simulink subsystem "EngineBasic_refsub"  (R2022a)
settings: Solver=VariableStepAuto  StartTime=0.0  StopTime=10.0  RelTol=1e-3
undefined symbols (not defined in the file): engine
libraries: fl_lib x11, nesl_utility x2, sdl_lib x1
settings Model: Creator=isaacito  LastModifiedBy=isaacito
settings SolverCC: AlgebraicLoopSolver=TrustRegion
settings DebuggingCC: UnconnectedInputMsg=warning  UnconnectedOutputMsg=warning  UnconnectedLineMsg=warning  SFMachineParentedDataDiag=warning
settings RTWCC: DLArmComputeVersion=19.05

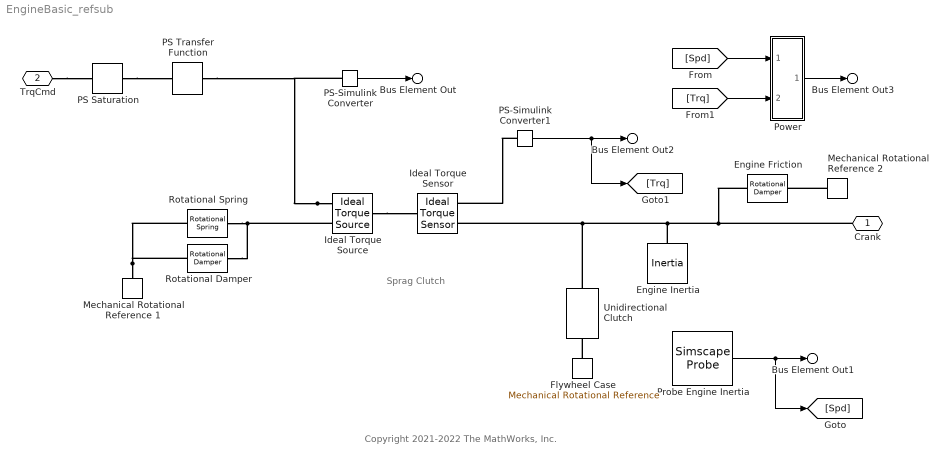
== system EngineBasic_refsub ==
  note: Copyright 2021-2022 The MathWorks, Inc.
  note: Sprag Clutch
  Engine Friction : fl_lib/Mechanical/Rotational Elements/Rotational Damper  D=engine.damping_Nm_per_rpm m*N/rpm  w_specify=off  w_priority=None  w=0 rad/s  w_nominal_specify=off  w_nominal_unit=rad/s  w_nominal_value=1  t_specify=off  t_priority=None  t=0 N*m  t_nominal_specify=off  t_nominal_unit=N*m  t_nominal_value=1
      settings: SourceProductBaseCode=PW,SS,VE
  Engine Inertia : fl_lib/Mechanical/Rotational Elements/Inertia  inertia=engine.inertia_kg_m2 kg*m^2  num_ports=foundation.enum.numPorts2.one  w_specify=on  w_priority=None  w=initial.engine_speed_rpm rpm  w_nominal_specify=off  w_nominal_unit=rad/s  w_nominal_value=1  t_specify=off  t_priority=None  t=0 N*m  t_nominal_specify=off  t_nominal_unit=N*m  t_nominal_value=1
      settings: SourceProductBaseCode=PW,SS,VE
      settings: AttributesFormatString=|
      | %<inertia> (%<inertia_unit>)
      | %<w> (%<w_unit>)
      | Priority: %<w_priority>
  Flywheel Case : fl_lib/Mechanical/Rotational Elements/Mechanical Rotational Reference
      settings: SourceProductBaseCode=PW,SS,VE
  Ideal Torque Sensor : fl_lib/Mechanical/Mechanical Sensors/Ideal Torque Sensor
      settings: SourceProductBaseCode=PW,SS,VE
  Ideal Torque Source : fl_lib/Mechanical/Mechanical Sources/Ideal Torque Source
      settings: SourceProductBaseCode=PW,SS,VE
  Mechanical Rotational Reference 1 : fl_lib/Mechanical/Rotational Elements/Mechanical Rotational Reference
      settings: SourceProductBaseCode=PW,SS,VE
  Mechanical Rotational Reference 2 : fl_lib/Mechanical/Rotational Elements/Mechanical Rotational Reference
      settings: SourceProductBaseCode=PW,SS,VE
  PS Saturation : fl_lib/Physical Signals/Nonlinear Operators/PS Saturation  upper_limit=engine.trqMax_Nm N*m  lower_limit=0 N*m
      settings: AttributesFormatString=%<upper_limit> (%<upper_limit_unit>)  SourceProductBaseCode=PW,SS,VE
  PS Transfer Function : fl_lib/Physical Signals/Linear Operators/PS Transfer Function  transfer_function_type=foundation.enum.transfer_function_type.lag  T=engine.lag_s s  T1=2 s  T2=1 s  y0=initial.engine_torque_Nm N*m
      settings: SourceProductBaseCode=PW,SS,VE  InternalSimscapePortConfiguration="{\"Bottom\":[],\"Left\":[{\"id\":\"U\",\"label\":\"\",\"type\":\"input\"}],\"Right\":[{\"id\":\"Y\",\"label\":\"\",\"type\":\"output\"}],\"Top\":[]}"
      settings: AttributesFormatString=|
      | %<T> [%<T_unit>]
      | Initial: %<y0> [%<y0_unit>]
  PS-Simulink Converter : nesl_utility/PS-Simulink Converter  PhysicalDomain=network_engine_domain  SubClassName=ps_output  LeftPortType=input  RightPortType=output  PseudoPeriodic=off  Frequencies=[]  VectorFormat=1-D array  Unit=N*m  AffineConversion=off
      settings: SourceProductBaseCode=SS,PW,VE
  PS-Simulink Converter1 : nesl_utility/PS-Simulink Converter  PhysicalDomain=network_engine_domain  SubClassName=ps_output  LeftPortType=input  RightPortType=output  PseudoPeriodic=off  Frequencies=[]  VectorFormat=1-D array  Unit=inherit  AffineConversion=off
      settings: SourceProductBaseCode=SS,PW,VE
  Power : Subsystem
  Probe Engine Inertia : SimscapeProbe  BoundBlock=2  Variables={w}
  Rotational Damper : fl_lib/Mechanical/Rotational Elements/Rotational Damper  D=engine.dampSpringFriction_Nm_per_rpm N*m/rpm  w_specify=off  w_priority=None  w=0 rad/s  w_nominal_specify=off  w_nominal_unit=rad/s  w_nominal_value=1  t_specify=off  t_priority=None  t=0 N*m  t_nominal_specify=off  t_nominal_unit=N*m  t_nominal_value=1
      settings: SourceProductBaseCode=PW,SS,VE
  Rotational Spring : fl_lib/Mechanical/Rotational Elements/Rotational Spring  spr_rate=engine.dampSpringStiffness_Nm_per_rad N*m/rad  w_specify=off  w_priority=None  w=0 rad/s  w_nominal_specify=off  w_nominal_unit=rad/s  w_nominal_value=1  t_specify=off  t_priority=None  t=0 N*m  t_nominal_specify=off  t_nominal_unit=N*m  t_nominal_value=1  phi_specify=on  phi_priority=Low  phi=0 rad  phi_nominal_specify=off  phi_nominal_unit=rad  phi_nominal_value=1
      settings: AttributesFormatString=Deformation priority: %<phi_priority>  SourceProductBaseCode=PW,SS,VE
  Unidirectional Clutch : sdl_lib/Clutches/Unidirectional Clutch  transmission_direction=2  initial_state_locked=sdl.enum.initial_lock.unlocked
      settings: AttributesFormatString=%<initial_state_locked>  SourceProductBaseCode=LD  InternalSimscapePortConfiguration="{\"Bottom\":[],\"Left\":[{\"id\":\"H\",\"label\":\"H\",\"type\":\"foundation.mechanical.rotational.rotational\"}],\"Right\":[{\"id\":\"R\",\"label\":\"R\",\"type\":\"foundation.mechanical.rotational.rotational\"}],\"Top\":[]}"
  Crank : PMIOPort  Side=Left
  TrqCmd : PMIOPort  Port=2  Side=Right
  Bus Element Out : Outport  PortName=Info  Element=EngTrqCmd
      settings: AttributesFormatString=%<Unit>
  Bus Element Out1 : Outport  PortName=Info  Element=EngSpd
      settings: AttributesFormatString=%<Unit>
  Bus Element Out2 : Outport  PortName=Info  Element=EngTrq
      settings: AttributesFormatString=%<Unit>
  Bus Element Out3 : Outport  PortName=Info  Element=EngPwr
      settings: AttributesFormatString=%<Unit>
  wires:
  Power/1(Pwr) -> Bus Element Out3/1
  [Trq] -> Power/2(Trq)
  [Spd] -> Power/1(Spd)
  PS-Simulink Converter1/1 -> [Trq], Bus Element Out2/1
  Probe Engine Inertia/1 -> [Spd], Bus Element Out1/1
  PS-Simulink Converter/1 -> Bus Element Out/1
  connections:
  Mechanical Rotational Reference 1/LConn1 -- Rotational Spring/LConn1 -- Rotational Damper/LConn1
  Rotational Spring/RConn1 -- Ideal Torque Source/RConn2 -- Rotational Damper/RConn1
  Ideal Torque Source/RConn1 -- PS Transfer Function/RConn1 -- PS-Simulink Converter/LConn1
  Crank/RConn1 -- Engine Inertia/LConn1 -- Unidirectional Clutch/LConn1 -- Ideal Torque Sensor/RConn1 -- Engine Friction/LConn1
  Flywheel Case/LConn1 -- Unidirectional Clutch/RConn1
  PS-Simulink Converter1/LConn1 -- Ideal Torque Sensor/RConn2
  Ideal Torque Source/LConn1 -- Ideal Torque Sensor/LConn1
  Mechanical Rotational Reference 2/LConn1 -- Engine Friction/RConn1
  TrqCmd/RConn1 -- PS Saturation/LConn1
  PS Saturation/RConn1 -- PS Transfer Function/LConn1

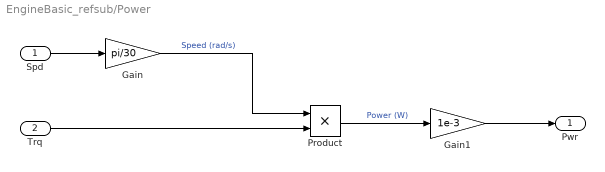
== system EngineBasic_refsub/Power ==
  Spd : Inport  Unit=rpm
  Trq : Inport  Port=2  Unit=N*m
  Gain : Gain  Gain=pi/30
  Gain1 : Gain  Gain=1e-3
  Product : Product
  Pwr : Outport  Unit=kW
  wires:
  Trq/1 -> Product/2
  Spd/1 -> Gain/1
  Gain/1 -> Product/1  "Speed (rad/s)"
  Product/1 -> Gain1/1  "Power (W)"
  Gain1/1 -> Pwr/1
